simulink model "Q1_sim"  (R2021a)
settings: Solver=VariableStepAuto  StartTime=0.0  StopTime=10.0  RelTol=1e-3
settings Model: Creator=sdjkhosh  LastModifiedBy=sdjkhosh

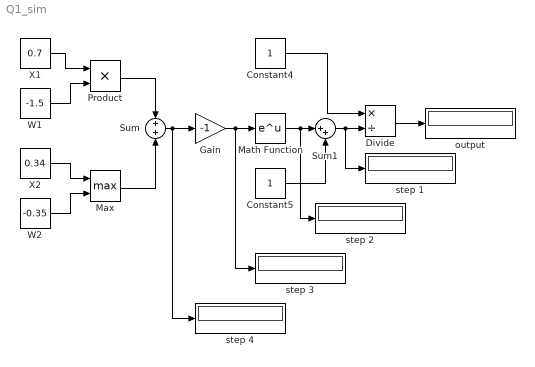
== system Q1_sim ==
  Constant4 : Constant
  Constant5 : Constant
  Divide : Product  Inputs=*/
  Gain : Gain  Gain=-1
  Math Function : Math  SaturateOnIntegerOverflow=on
  Max : MinMax  Function=max  Inputs=2
  Product : Product
  Sum : Sum
  Sum1 : Sum  Inputs=|++
  W1 : Constant  Value=-1.5
  W2 : Constant  Value=-0.35
  X1 : Constant  Value=0.7
  X2 : Constant  Value=0.34
  output : Display
  step {1..4} (4 alike) : Display
  wires:
  X1/1 -> Product/1
  W1/1 -> Product/2
  X2/1 -> Max/1
  W2/1 -> Max/2
  Product/1 -> Sum/1
  Max/1 -> Sum/2
  Sum/1 -> step 4/1, Gain/1
  Gain/1 -> step 3/1, Math Function/1
  Math Function/1 -> step 2/1, Sum1/1
  Constant5/1 -> Sum1/2
  Sum1/1 -> step 1/1, Divide/2
  Constant4/1 -> Divide/1
  Divide/1 -> output/1
